simulink model "halleffect_pos_filter"  (R2022a)
settings: Solver=FixedStepDiscrete  StartTime=0.0  StopTime=10  FixedStep=0.0001  RelTol=1e-3
undefined symbols (not defined in the file): DiscIntNeverNeededParam
libraries: dspswit3 x1, simulink x1
settings Model: Creator=EEED Stores 381  LastModifiedBy=EEED Stores 381

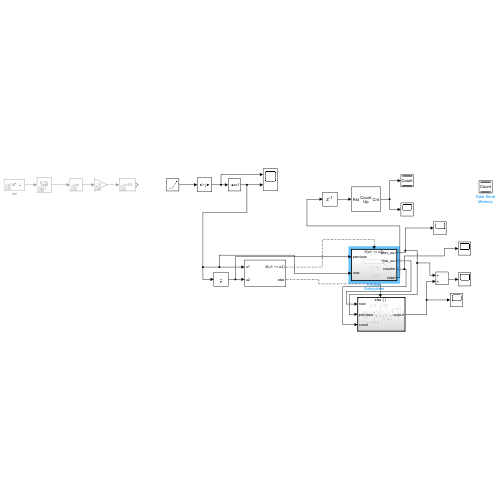
[thumbnail: Simulink's stored preview of the top-level diagram]
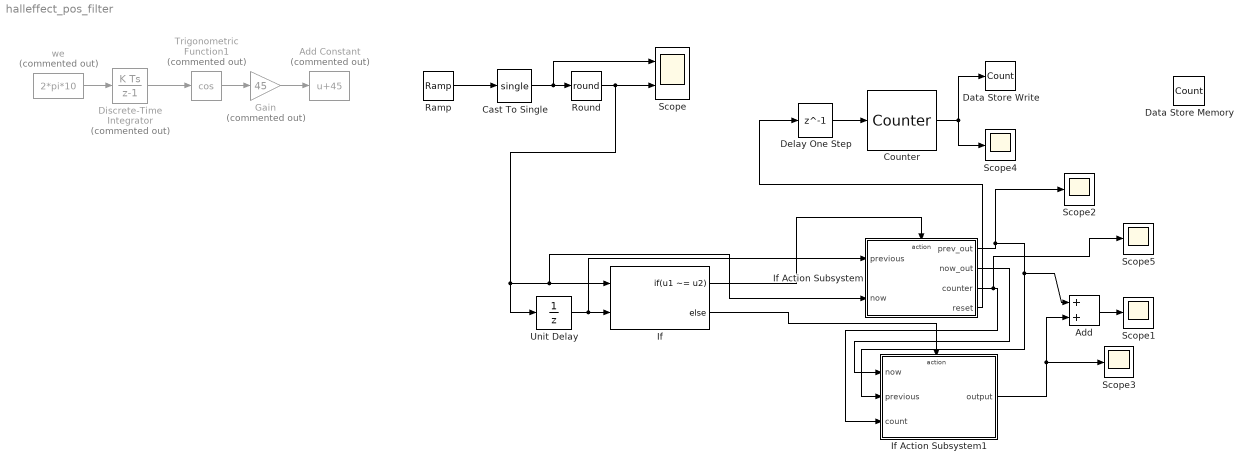
== system halleffect_pos_filter ==
  Add : Sum
  Add Constant : Bias  Commented=on  Bias=45  SaturateOnIntegerOverflow=off
  Cast To Single : DataTypeConversion  OutDataTypeStr=single  SaturateOnIntegerOverflow=off  RndMeth=Floor
  Counter : dspswit3/Counter  Direction=Up  CountEvent=Free running  CounterSize=32 bits  MaxCount=255  InitialCount=0  Output=Count  HitValue=32  ResetInput=on  SamplesPerFrame=1  Ts=-1  CntDtype=single  HitDtype=Logical
  Data Store Memory : DataStoreMemory  DataStoreName=Count  WriteAfterWriteMsg=warning  ShowAdditionalParam=off
  Data Store Write : DataStoreWrite  DataStoreName=Count  IndexOptions=Index vector (dialog)  Indices=1  OutputSizes=1
  Delay One Step : Delay  DelayLength=1
  Discrete-Time Integrator : DiscreteIntegrator  Commented=on  SampleTime=-1  ICPrevOutput=DiscIntNeverNeededParam  ICPrevScaledInput=DiscIntNeverNeededParam
  Gain : Gain  Commented=on  Gain=45
  If : If  NumInputs=2  IfExpression=u1 ~= u2
  If Action Subsystem : Subsystem  TreatAsAtomicUnit=on
  If Action Subsystem1 : Subsystem  TreatAsAtomicUnit=on
  Ramp : simulink/Sources/Ramp  slope=5  start=0  InitialOutput=0
  Round : Rounding  Operator=round
  Scope : Scope  NumInputPorts=2
  Scope{1..5} (5 alike) : Scope
  Trigonometric Function1 : Trigonometry  Commented=on  Operator=cos
  Unit Delay : UnitDelay  SampleTime=-1  HasFrameUpgradeWarning=on
  we : Constant  Commented=on  Value=2*pi*10  SampleTime=-1
  wires:
  Gain/1 -> Add Constant/1
  Round/1 -> Scope/2, Unit Delay/1, If Action Subsystem/2(now), If/1
  Discrete-Time Integrator/1 -> Trigonometric Function1/1
  we/1 -> Discrete-Time Integrator/1
  Trigonometric Function1/1 -> Gain/1
  Unit Delay/1 -> If Action Subsystem/1(previous), If/2
  If/1 -> If Action Subsystem/Action
  Cast To Single/1 -> Scope/1, Round/1
  If/2 -> If Action Subsystem1/Action
  If Action Subsystem/1(prev_out) -> Scope2/1, If Action Subsystem1/2(previous), Add/1
  If Action Subsystem/2(now_out) -> If Action Subsystem1/1(now)
  If Action Subsystem1/1(output) -> Scope3/1, Add/2
  Ramp/1 -> Cast To Single/1
  Add/1 -> Scope1/1
  Counter/1 -> Scope4/1, Data Store Write/1
  If Action Subsystem/3(counter) -> Scope5/1, If Action Subsystem1/3(count)
  If Action Subsystem/4(reset) -> Delay One Step/1
  Delay One Step/1 -> Counter/1

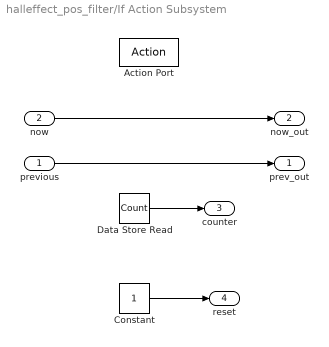
== system halleffect_pos_filter/If Action Subsystem ==
  previous : Inport
  now : Inport  Port=2
  Action Port : ActionPort  InitializeStates=reset  ActionPortLabel=if(u1 ~= u2)
  Constant : Constant
  Data Store Read : DataStoreRead  DataStoreName=Count  IndexOptions=Index vector (dialog)  Indices=1  OutputSizes=1
  prev_out : Outport
  now_out : Outport  Port=2
  counter : Outport  Port=3
  reset : Outport  Port=4  OutputWhenDisabled=reset  InitialOutput=0
  wires:
  previous/1 -> prev_out/1
  now/1 -> now_out/1
  Data Store Read/1 -> counter/1
  Constant/1 -> reset/1

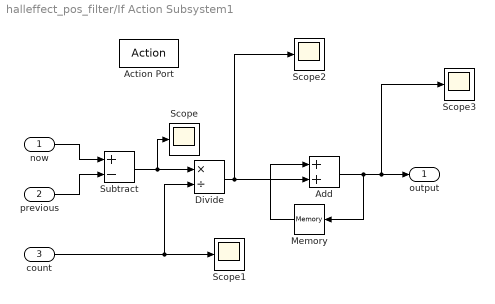
== system halleffect_pos_filter/If Action Subsystem1 ==
  now : Inport
  previous : Inport  Port=2
  count : Inport  Port=3
  Action Port : ActionPort  ActionPortLabel=else
  Add : Sum
  Divide : Product  Inputs=*/  RndMeth=Zero  SaturateOnIntegerOverflow=on
  Memory : Memory  InheritSampleTime=on  LinearizeAsDelay=on
  Scope{,1..3} (4 alike) : Scope
  Subtract : Sum  Inputs=+-
  output : Outport  InitialOutput=0
  wires:
  now/1 -> Subtract/1
  previous/1 -> Subtract/2
  Subtract/1 -> Scope/1, Divide/1
  count/1 -> Divide/2, Scope1/1
  Divide/1 -> Add/2, Scope2/1
  Memory/1 -> Add/1
  Add/1 -> Memory/1, Scope3/1, output/1
